simulink model "sampleModel365"  (R2021b)
settings: Solver=VariableStepAuto  StartTime=0.0  StopTime=10.0  RelTol=1e-3
undefined symbols (not defined in the file or in its folder): DiscIntNeverNeededParam
libraries: simulink x9, slpidlib x4
settings Model: Creator=user  LastModifiedBy=user

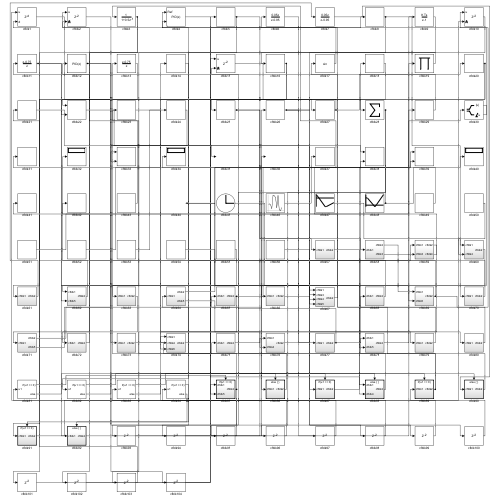
[thumbnail: Simulink's stored preview of the top-level diagram]
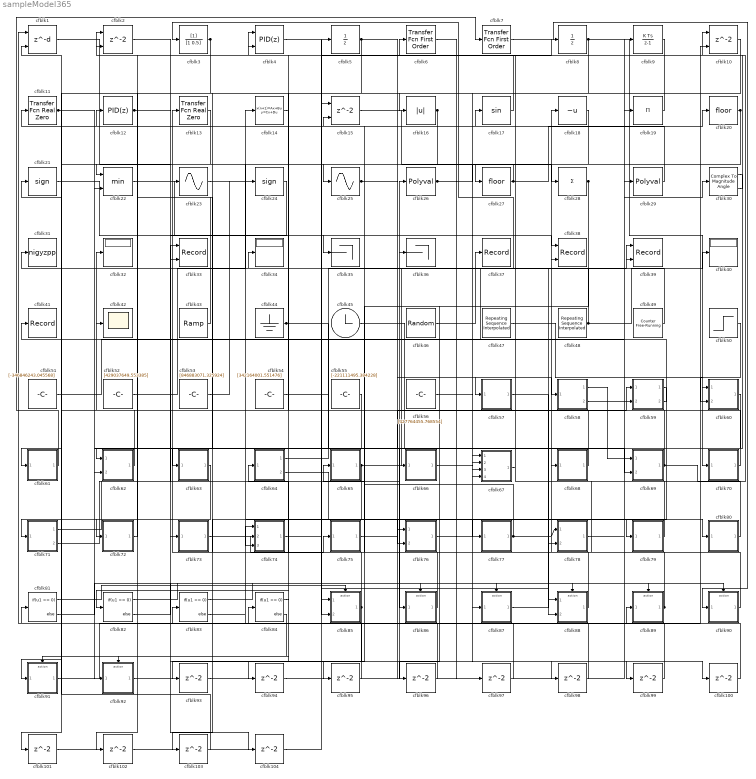
== system sampleModel365 ==
  cfblk1 : Delay  DelayLengthSource=Input port  SampleTime=1
      settings: InputPortMap=u0,p1
  cfblk10 : Delay  ShowEnablePort=on  SampleTime=1
      settings: InputPortMap=u0,e6
  cfblk{93..104} (12 alike) : Delay  SampleTime=1
  cfblk11 : simulink/Discrete/Transfer Fcn Real Zero  ZeroZ=0.75  ICPrevInput=0.0  DoSatur=off
      settings: SourceProductBaseCode=SL
  cfblk12 : slpidlib/PID Controller  Controller=PID  Form=Parallel  TimeDomain=Discrete-time  UseExternalTs=off  SampleTime=1  IntegratorMethod=Forward Euler  FilterMethod=Forward Euler  ControllerParametersSource=internal  P=1  I=1  D=0  UseFilter=on  N=100  TunerSelectOption=Transfer Function Based (PID Tuner App)  InitialConditionSource=internal  InitialConditionForIntegrator=0  InitialConditionForFilter=0  DifferentiatorICPrevScaledInput=0  ExternalReset=none  TrackingMode=off  Kt=1  LimitOutput=off  SatLimitsSource=internal  UpperSaturationLimit=inf  LowerSaturationLimit=-inf  LinearizeAsGain=off  AntiWindupMode=none  Kb=1  POutMin=[]  POutMax=[]  IOutMin=[]  IOutMax=[]  DOutMin=[]  DOutMax=[]  NOutMin=[]  NOutMax=[]  SumOutMin=[]  SumOutMax=[]  SaturationOutMin=[]  SaturationOutMax=[]  PParamMin=[]  PParamMax=[]  IParamMin=[]  IParamMax=[]  DParamMin=[]  DParamMax=[]  NParamMin=[]  NParamMax=[]  KbParamMin=[]  KbParamMax=[]  KtParamMin=[]  KtParamMax=[]  KbOutMin=[]  KbOutMax=[]  KtOutMin=[]  KtOutMax=[]  IntegratorOutMin=[]  IntegratorOutMax=[]  FilterOutMin=[]  FilterOutMax=[]  SumI1OutMin=[]  SumI1OutMax=[]  SumI2OutMin=[]  SumI2OutMax=[]  SumI3OutMin=[]  SumI3OutMax=[]  SumI4OutMin=[]  SumI4OutMax=[]  SumDOutMin=[]  SumDOutMax=[]  DifferentiatorOutMin=[]  DifferentiatorOutMax=[]  FilterDiffOutCoefMin=[]  FilterDiffOutCoefMax=[]  ReciprocalOutMin=[]  ReciprocalOutMax=[]  SumDenOutMin=[]  SumDenOutMax=[]  SumNumOutMin=[]  SumNumOutMax=[]  DivideOutMin=[]  DivideOutMax=[]  UdiffTsProdOutMin=[]  UdiffTsProdOutMax=[]  NTsProdOutMin=[]  NTsProdOutMax=[]  UintegralTsProdOutMin=[]  UintegralTsProdOutMax=[]  UngainTsProdOutMin=[]  UngainTsProdOutMax=[]  IntegratorContinuousStateAttributes=''  IntegratorStateMustResolveToSignalObject=off  IntegratorRTWStateStorageClass=Auto  FilterContinuousStateAttributes=''  FilterStateMustResolveToSignalObject=off  FilterRTWStateStorageClass=Auto  ParallelPVariant=InternalParameters  IdealPVariant=Disabled  IVariant=InternalParameters  DVariant=InternalParameters  IntegratorVariant=Discrete  SatVariant=Disabled  AWVariant=Passthrough  PCopyVariant=Disabled  TRVariant=Disabled  FdbkBlocksVariant=Forward  IdealPFdbkVariant=Disabled  SatFdbkVariant=Disabled  DerivativeFilterVariant=ForwardEulerFilter  NVariant=InternalParameters  NCopyVariant=Disabled  FilterICVariant=InternalICsFilter  IntegratorICVariant=InternalICs  ExternalResetVariant=Disabled  TRSumVariant=Passthrough  SumFdbkVariant=Disabled  SumVariant=Sum_PID  TsampFilterVariant=InternalTs  TsampNgainVariant=Passthrough  TsampIntegralVariant=Passthrough  ExternalSaturationOutDataTypeStr=Inherit: Same as second input
  cfblk13 : simulink/Discrete/Transfer Fcn Real Zero  ZeroZ=0.75  ICPrevInput=0.0  DoSatur=off
      settings: SourceProductBaseCode=SL
  cfblk14 : DiscreteStateSpace
  cfblk15 : Delay  ShowEnablePort=on  SampleTime=1
      settings: InputPortMap=u0,e6
  cfblk16 : Abs
  cfblk17 : Trigonometry
  cfblk18 : UnaryMinus
  cfblk19 : Product  Inputs=*
  cfblk2 : Delay  ShowEnablePort=on  SampleTime=1
      settings: InputPortMap=u0,e6
  cfblk20 : Rounding
  cfblk21 : Signum
  cfblk22 : MinMax  Inputs=2
  cfblk23 : Sin  TimeSource=Use external signal  SampleTime=0
  cfblk24 : Signum
  cfblk25 : Sin  TimeSource=Use external signal  SampleTime=0
  cfblk26 : Polyval  Coefs=[ +2.081618890e-019, -1.441693666e-014, +4.719686976e-010, -8.536869453e-006, +1.621573104e-001, -8.087801117e+001 ]
  cfblk27 : Rounding
  cfblk28 : Sum  Inputs=+
  cfblk29 : Polyval  Coefs=[ +2.081618890e-019, -1.441693666e-014, +4.719686976e-010, -8.536869453e-006, +1.621573104e-001, -8.087801117e+001 ]
  cfblk3 : DiscreteFilter  SampleTime=1
  cfblk30 : ComplexToMagnitudeAngle
  cfblk31 : ToWorkspace  VariableName=nigyzpp  SaveFormat=Timeseries  SampleTime=-1
  cfblk32 : Display
  cfblk33 : Record  FileSettingsInternal="{\"entries\":[{\"content\":{\"excelSettings\":{\"content\":{},\"type\":\"Streamout.ExcelSettings\"}},\"type\":\"Streamout.FileSettingStorage\",\"uuid\":\"567b8140-eb5c-4048-b530-8f92b88b9877\"}],\"packageUris\":[\"http://schema.mathworks.com/mf0/streamout_blocks/R2020a\"],\"version\":\"1.0\"}"  Layout=[1 1]  SignalsInternal="{\"entries\":[{\"content\":{\"signals\":[{\"content\":{\"blockPath\":[\"sampleModel365/cfblk33\"],\"channel\":[],\"dimensions\":[1],\"domain\":\"sampleModel365/cfblk33\",\"lineColor\":\"#a2142f\",\"plots\":[1],\"port\":1,\"sid\":[\"\"],\"signalID\":15095,\"signalName\":\"cfblk71:1\"},\"type\":\"RecordBlkView.Signal\",\"uuid\":\"13d7f1e2-b6fb-48eb-b80d-9a015310c975\"},{\"content\":{\"blockPath\":[\"sampleModel365/cfblk33\"],\"channel\":[],\"dimensions\":[1],\"domain\":\"sampleModel365/cfblk33\",\"lineColor\":\"#139fff\",\"plots\":[1],\"port\":2,\"sid\":[\"\"],\"signalID\":15099,\"signalName\":\"cfblk24\"},\"type\":\"RecordBlkView.Signal\",\"uuid\":\"a06a9fc9-9345-432e-829d-64d9e5ba65b8\"}]},\"type\":\"RecordBlkView.InputSignals\",\"uuid\":\"33d499b8-4f10-4db5-961c-bad95c7f5677\"}],\"packageUris\":[\"http://schema.mathworks.com/mf0/streamout_blocks/R2020a\"],\"version\":\"1.0\"}"  VisualizationBindings="{\"xyplotplugin\":{\"info\":[{\"series\":[{\"bindingParametersList\":[{\"parameter\":\"X-Axis\",\"signalID\":15095,\"signalName\":\"cfblk71:1\"},{\"parameter\":\"Y-Axis\",\"signalID\":15099,\"signalName\":\"cfblk24\"}],\"seriesID\":36555}],\"subplotID\":1}]}}"  CompatibilityTag=XY
  cfblk34 : Display
  cfblk35 : Terminator
  cfblk36 : Terminator
  cfblk37 : Record  FileSettingsInternal="{\"entries\":[{\"content\":{\"excelSettings\":{\"content\":{},\"type\":\"Streamout.ExcelSettings\"}},\"type\":\"Streamout.FileSettingStorage\",\"uuid\":\"649bd7b5-baee-4403-bfdf-0451a9d50882\"}],\"packageUris\":[\"http://schema.mathworks.com/mf0/streamout_blocks/R2020a\"],\"version\":\"1.0\"}"  SignalsInternal="{\"entries\":[{\"content\":{\"signals\":[{\"content\":{\"blockPath\":[\"sampleModel365/cfblk37\"],\"channel\":[],\"dimensions\":[1],\"domain\":\"sampleModel365/cfblk37\",\"lineColor\":\"#22b573\",\"plots\":[1],\"port\":1,\"sid\":[\"\"],\"signalID\":15119,\"signalName\":\"cfblk46\"},\"type\":\"RecordBlkView.Signal\",\"uuid\":\"1a7fcce6-5cc4-4007-aa49-3d2bea6aa8b4\"}]},\"type\":\"RecordBlkView.InputSignals\",\"uuid\":\"0982ba8e-6094-4d7a-b36e-3969a046187e\"}],\"packageUris\":[\"http://schema.mathworks.com/mf0/streamout_blocks/R2020a\"],\"version\":\"1.0\"}"  VisualizationBindings="{\"sparklinesplugin\":{\"info\":[{\"bindingParametersList\":[],\"subplotID\":1}]}}"
  cfblk38 : Record  FileSettingsInternal="{\"entries\":[{\"content\":{\"excelSettings\":{\"content\":{},\"type\":\"Streamout.ExcelSettings\"}},\"type\":\"Streamout.FileSettingStorage\",\"uuid\":\"1ff4d437-0c84-40b7-91d9-f5fc12d76050\"}],\"packageUris\":[\"http://schema.mathworks.com/mf0/streamout_blocks/R2020a\"],\"version\":\"1.0\"}"  Layout=[1 1]  SignalsInternal="{\"entries\":[{\"content\":{\"signals\":[{\"content\":{\"blockPath\":[\"sampleModel365/cfblk38\"],\"channel\":[],\"dimensions\":[1],\"domain\":\"sampleModel365/cfblk38\",\"lineColor\":\"#a2142f\",\"plots\":[1],\"port\":1,\"sid\":[\"\"],\"signalID\":15103,\"signalName\":\"cfblk22\"},\"type\":\"RecordBlkView.Signal\",\"uuid\":\"a984cc03-4ad2-4885-a72c-2beb6033d68e\"},{\"content\":{\"blockPath\":[\"sampleModel365/cfblk38\"],\"channel\":[],\"dimensions\":[1],\"domain\":\"sampleModel365/cfblk38\",\"lineColor\":\"#139fff\",\"plots\":[1],\"port\":2,\"sid\":[\"\"],\"signalID\":15123,\"signalName\":\"cfblk44\"},\"type\":\"RecordBlkView.Signal\",\"uuid\":\"cf2bfc31-ea28-4664-8696-6d3ddec068b2\"}]},\"type\":\"RecordBlkView.InputSignals\",\"uuid\":\"835b0b7a-af76-47df-882f-258c594722fd\"}],\"packageUris\":[\"http://schema.mathworks.com/mf0/streamout_blocks/R2020a\"],\"version\":\"1.0\"}"  VisualizationBindings="{\"xyplotplugin\":{\"info\":[{\"series\":[{\"bindingParametersList\":[{\"parameter\":\"X-Axis\",\"signalID\":15103,\"signalName\":\"cfblk22\"},{\"parameter\":\"Y-Axis\",\"signalID\":15123,\"signalName\":\"cfblk44\"}],\"seriesID\":61757}],\"subplotID\":1}]}}"  CompatibilityTag=XY
  cfblk39 : Record  FileSettingsInternal="{\"entries\":[{\"content\":{\"excelSettings\":{\"content\":{},\"type\":\"Streamout.ExcelSettings\"}},\"type\":\"Streamout.FileSettingStorage\",\"uuid\":\"35b5ed4a-cb0b-4459-8fb2-d4d30692ccee\"}],\"packageUris\":[\"http://schema.mathworks.com/mf0/streamout_blocks/R2020a\"],\"version\":\"1.0\"}"  Layout=[1 1]  SignalsInternal="{\"entries\":[{\"content\":{\"signals\":[{\"content\":{\"blockPath\":[\"sampleModel365/cfblk39\"],\"channel\":[],\"dimensions\":[1],\"domain\":\"sampleModel365/cfblk39\",\"lineColor\":\"#a2142f\",\"plots\":[1],\"port\":1,\"sid\":[\"\"],\"signalID\":15107,\"signalName\":\"cfblk65\"},\"type\":\"RecordBlkView.Signal\",\"uuid\":\"c0428a1b-d602-48ef-ba58-3bcf674a13e3\"},{\"content\":{\"blockPath\":[\"sampleModel365/cfblk39\"],\"channel\":[],\"dimensions\":[1],\"domain\":\"sampleModel365/cfblk39\",\"lineColor\":\"#139fff\",\"plots\":[1],\"port\":2,\"sid\":[\"\"],\"signalID\":15111,\"signalName\":\"cfblk87\"},\"type\":\"RecordBlkView.Signal\",\"uuid\":\"106950b7-24c9-4dcc-9644-3f44a9cb415d\"}]},\"type\":\"RecordBlkView.InputSignals\",\"uuid\":\"4c517a09-619e-4c48-972b-e804149b64f6\"}],\"packageUris\":[\"http://schema.mathworks.com/mf0/streamout_blocks/R2020a\"],\"version\":\"1.0\"}"  VisualizationBindings="{\"xyplotplugin\":{\"info\":[{\"series\":[{\"bindingParametersList\":[{\"parameter\":\"X-Axis\",\"signalID\":15107,\"signalName\":\"cfblk65\"},{\"parameter\":\"Y-Axis\",\"signalID\":15111,\"signalName\":\"cfblk87\"}],\"seriesID\":63832}],\"subplotID\":1}]}}"  CompatibilityTag=XY
  cfblk4 : slpidlib/PID Controller (2DOF)  Controller=PID  Form=Parallel  TimeDomain=Discrete-time  UseExternalTs=off  SampleTime=1  IntegratorMethod=Forward Euler  FilterMethod=Forward Euler  ControllerParametersSource=internal  P=1  I=1  D=0  UseFilter=on  N=100  b=1  c=1  TunerSelectOption=Transfer Function Based (PID Tuner App)  InitialConditionSource=internal  InitialConditionForIntegrator=0  InitialConditionForFilter=0  DifferentiatorICPrevScaledInput=0  ExternalReset=none  TrackingMode=off  Kt=1  LimitOutput=off  SatLimitsSource=internal  UpperSaturationLimit=inf  LowerSaturationLimit=-inf  LinearizeAsGain=off  AntiWindupMode=none  Kb=1  POutMin=[]  POutMax=[]  IOutMin=[]  IOutMax=[]  DOutMin=[]  DOutMax=[]  NOutMin=[]  NOutMax=[]  bOutMin=[]  bOutMax=[]  cOutMin=[]  cOutMax=[]  SumOutMin=[]  SumOutMax=[]  SaturationOutMin=[]  SaturationOutMax=[]  PParamMin=[]  PParamMax=[]  IParamMin=[]  IParamMax=[]  DParamMin=[]  DParamMax=[]  NParamMin=[]  NParamMax=[]  bParamMin=[]  bParamMax=[]  cParamMin=[]  cParamMax=[]  KbParamMin=[]  KbParamMax=[]  KtParamMin=[]  KtParamMax=[]  KbOutMin=[]  KbOutMax=[]  KtOutMin=[]  KtOutMax=[]  IntegratorOutMin=[]  IntegratorOutMax=[]  FilterOutMin=[]  FilterOutMax=[]  SumI1OutMin=[]  SumI1OutMax=[]  SumI2OutMin=[]  SumI2OutMax=[]  SumI3OutMin=[]  SumI3OutMax=[]  SumI4OutMin=[]  SumI4OutMax=[]  SumDOutMin=[]  SumDOutMax=[]  Sum1OutMin=[]  Sum1OutMax=[]  Sum2OutMin=[]  Sum2OutMax=[]  Sum3OutMin=[]  Sum3OutMax=[]  DifferentiatorOutMin=[]  DifferentiatorOutMax=[]  FilterDiffOutCoefMin=[]  FilterDiffOutCoefMax=[]  ReciprocalOutMin=[]  ReciprocalOutMax=[]  SumDenOutMin=[]  SumDenOutMax=[]  SumNumOutMin=[]  SumNumOutMax=[]  DivideOutMin=[]  DivideOutMax=[]  UdiffTsProdOutMin=[]  UdiffTsProdOutMax=[]  NTsProdOutMin=[]  NTsProdOutMax=[]  UintegralTsProdOutMin=[]  UintegralTsProdOutMax=[]  UngainTsProdOutMin=[]  UngainTsProdOutMax=[]  IntegratorContinuousStateAttributes=''  IntegratorStateMustResolveToSignalObject=off  IntegratorRTWStateStorageClass=Auto  FilterContinuousStateAttributes=''  FilterStateMustResolveToSignalObject=off  FilterRTWStateStorageClass=Auto  ParallelPVariant=InternalParameters  IdealPVariant=Disabled  IVariant=InternalParameters  DVariant=InternalParameters  bVariant=InternalParameters  cVariant=InternalParameters  IntegratorVariant=Discrete  SatVariant=Disabled  AWVariant=Passthrough  PCopyVariant=Disabled  TRVariant=Disabled  FdbkBlocksVariant=Forward  IdealPFdbkVariant=Disabled  SatFdbkVariant=Disabled  DerivativeFilterVariant=ForwardEulerFilter  NVariant=InternalParameters  NCopyVariant=Disabled  FilterICVariant=InternalICsFilter  IntegratorICVariant=InternalICs  ExternalResetVariant=Disabled  TRSumVariant=Passthrough  SumFdbkVariant=Disabled  SumVariant=Sum_PID  TsampFilterVariant=InternalTs  TsampNgainVariant=Passthrough  TsampIntegralVariant=Passthrough  ExternalSaturationOutDataTypeStr=Inherit: Same as second input
      settings: SourceProductBaseCode=SL
  cfblk40 : Display
  cfblk41 : Record  FileSettingsInternal="{\"entries\":[{\"content\":{\"excelSettings\":{\"content\":{},\"type\":\"Streamout.ExcelSettings\"}},\"type\":\"Streamout.FileSettingStorage\",\"uuid\":\"5481fc23-8463-4565-9524-5e1ed1cb160f\"}],\"packageUris\":[\"http://schema.mathworks.com/mf0/streamout_blocks/R2020a\"],\"version\":\"1.0\"}"  SignalsInternal="{\"entries\":[{\"content\":{\"signals\":[{\"content\":{\"blockPath\":[\"sampleModel365/cfblk41\"],\"channel\":[],\"dimensions\":[1],\"domain\":\"sampleModel365/cfblk41\",\"lineColor\":\"#fe330a\",\"plots\":[1],\"port\":1,\"sid\":[\"\"],\"signalID\":15115,\"signalName\":\"cfblk59:2\"},\"type\":\"RecordBlkView.Signal\",\"uuid\":\"222ed1ed-24d6-4460-972e-87adfa1e83d3\"}]},\"type\":\"RecordBlkView.InputSignals\",\"uuid\":\"1feaa0a2-3980-4dbe-9ab3-42cb594308e1\"}],\"packageUris\":[\"http://schema.mathworks.com/mf0/streamout_blocks/R2020a\"],\"version\":\"1.0\"}"  VisualizationBindings="{\"sparklinesplugin\":{\"info\":[{\"bindingParametersList\":[],\"subplotID\":1}]}}"
  cfblk42 : Scope
  cfblk43 : simulink/Sources/Ramp  slope=[2383.054350]  start=[44.880096]  InitialOutput=[485045.496723]
  cfblk44 : Ground
  cfblk45 : Clock
  cfblk46 : RandomNumber  Mean=[75307.969094]  Variance=[43913.906071]  Seed=[27084174.000000]  SampleTime=0.1
  cfblk47 : simulink/Sources/Repeating Sequence Interpolated  OutValues=[324115040.329646, 113958309.694816, -785240119.694534, -752060174.629684, -422976193.941777]  TimeValues=[0 0.1 0.5 0.6 1].'  LookUpMeth=Use Input Nearest  tsamp=0.01  OutMin=[]  OutMax=[]  OutDataTypeStr=double  OutputDataTypeScalingMode=double  OutDataType=fixdt(0,8)  OutScaling=2^-10
  cfblk48 : simulink/Sources/Repeating Sequence Interpolated  OutValues=[666690424.086203, 616793045.343907, -127611017.511921, 16668326.026093, 946909106.545576]  TimeValues=[0 0.1 0.5 0.6 1].'  LookUpMeth=Use Input Below  tsamp=0.01  OutMin=[]  OutMax=[]  OutDataTypeStr=double  OutputDataTypeScalingMode=double  OutDataType=fixdt(0,8)  OutScaling=2^-10
  cfblk49 : simulink/Sources/Counter Free-Running  NumBits=[29.000000]  tsamp=-1
  cfblk5 : UnitDelay  HasFrameUpgradeWarning=on
  cfblk50 : Step  Time=[41.000000]  Before=[181754476.570915]  After=[944807555.087493]  SampleTime=0
  cfblk51 : Constant  Value=[-346846243.045568]  SampleTime=1
  cfblk52 : Constant  Value=[429037649.553385]  SampleTime=1
  cfblk53 : Constant  Value=[846883071.325924]  SampleTime=1
  cfblk54 : Constant  Value=[342164001.551476]  SampleTime=1
  cfblk55 : Constant  Value=[-221111495.384228]  SampleTime=1
  cfblk56 : Constant  Value=[427764455.768554]  SampleTime=1
  cfblk57 : Subsystem
  cfblk58 : Subsystem
  cfblk59 : Subsystem
  cfblk6 : simulink/Discrete/Transfer Fcn First Order  PoleZ=0.95  ICPrevOutput=0.0  DoSatur=off
  cfblk60 : Subsystem
  cfblk61 : Subsystem
  cfblk62 : Subsystem
  cfblk63 : Subsystem
  cfblk64 : Subsystem
  cfblk65 : Subsystem
  cfblk66 : Subsystem
  cfblk67 : Subsystem
  cfblk68 : Subsystem
  cfblk69 : Subsystem
  cfblk7 : simulink/Discrete/Transfer Fcn First Order  PoleZ=0.95  ICPrevOutput=0.0  DoSatur=off
  cfblk70 : Subsystem
  cfblk71 : Subsystem
  cfblk72 : Subsystem
  cfblk73 : Subsystem
  cfblk74 : Subsystem
  cfblk75 : Subsystem
  cfblk76 : Subsystem
  cfblk77 : Subsystem
  cfblk78 : Subsystem
  cfblk79 : Subsystem
  cfblk8 : UnitDelay  HasFrameUpgradeWarning=on
  cfblk80 : Subsystem
  cfblk{81..84} (4 alike) : If  IfExpression=u1 >= 0  SampleTime=1
  cfblk85 : Subsystem  TreatAsAtomicUnit=on
  cfblk86 : Subsystem  TreatAsAtomicUnit=on
  cfblk87 : Subsystem  TreatAsAtomicUnit=on
  cfblk88 : Subsystem  TreatAsAtomicUnit=on
  cfblk89 : Subsystem  TreatAsAtomicUnit=on
  cfblk9 : DiscreteIntegrator  ICPrevOutput=DiscIntNeverNeededParam  ICPrevScaledInput=DiscIntNeverNeededParam
  cfblk90 : Subsystem  TreatAsAtomicUnit=on
  cfblk91 : Subsystem  TreatAsAtomicUnit=on
  cfblk92 : Subsystem  TreatAsAtomicUnit=on
  wires:
  cfblk89/1(cfblk2) -> cfblk18/1, cfblk68/1(cfblk1)
  cfblk14/1 -> cfblk82/1
  cfblk6/1 -> cfblk77/1(cfblk1)
  cfblk46/1 -> cfblk37/1
  cfblk47/1 -> cfblk70/1(cfblk1)
  cfblk92/1(cfblk2) -> cfblk26/1
  cfblk53/1 -> cfblk24/1
  cfblk67/1(cfblk2) -> cfblk3/1
  cfblk85/1(cfblk2) -> cfblk13/1, cfblk103/1
  cfblk3/1 -> cfblk22/1, cfblk72/1(cfblk1)
  cfblk25/1 -> cfblk58/1(cfblk1), cfblk67/4(cfblk5)
  cfblk5/1 -> cfblk63/1(cfblk1), cfblk57/1(cfblk1)
  cfblk1/1 -> cfblk73/1(cfblk1)
  cfblk58/1(cfblk2) -> cfblk69/1(cfblk1)
  cfblk30/1 -> cfblk62/1(cfblk1)
  cfblk54/1 -> cfblk69/2(cfblk5)
  cfblk60/1(cfblk2) -> cfblk86/1(cfblk1)
  cfblk15/1 -> cfblk27/1
  cfblk55/1 -> cfblk62/2(cfblk5)
  cfblk48/1 -> cfblk34/1, cfblk40/1
  cfblk71/1(cfblk2) -> cfblk33/1
  cfblk71/2(cfblk5) -> cfblk36/1
  cfblk69/1(cfblk2) -> cfblk10/1, cfblk12/1
  cfblk70/1(cfblk2) -> cfblk32/1
  cfblk65/1(cfblk2) -> cfblk39/1, cfblk93/1
  cfblk57/1(cfblk2) -> cfblk88/1(cfblk1)
  cfblk87/1(cfblk2) -> cfblk39/2
  cfblk29/1 -> cfblk17/1
  cfblk23/1 -> cfblk76/2(cfblk4)
  cfblk19/1 -> cfblk16/1
  cfblk49/1 -> cfblk31/1
  cfblk26/1 -> cfblk28/1, cfblk97/1, cfblk98/1
  cfblk21/1 -> cfblk67/1(cfblk1)
  cfblk56/1 -> cfblk87/1(cfblk1)
  cfblk7/1 -> cfblk90/1(cfblk1)
  cfblk18/1 -> cfblk22/2
  cfblk27/1 -> cfblk20/1, cfblk25/1
  cfblk22/1 -> cfblk38/1
  cfblk17/1 -> cfblk6/1
  cfblk4/1 -> cfblk88/2(cfblk4)
  cfblk30/2 -> cfblk4/1
  cfblk91/1(cfblk2) -> cfblk10/2
  cfblk28/1 -> cfblk95/1, cfblk96/1
  cfblk68/1(cfblk2) -> cfblk4/2
  cfblk8/1 -> cfblk60/1(cfblk1), cfblk61/1(cfblk1)
  cfblk44/1 -> cfblk38/2, cfblk67/3(cfblk4)
  cfblk76/1(cfblk2) -> cfblk80/1(cfblk1)
  cfblk62/1(cfblk2) -> cfblk21/1
  cfblk73/1(cfblk2) -> cfblk75/1(cfblk1)
  cfblk75/1(cfblk2) -> cfblk59/1(cfblk1)
  cfblk78/1(cfblk2) -> cfblk9/1
  cfblk43/1 -> cfblk2/1
  cfblk79/1(cfblk2) -> cfblk11/1
  cfblk88/1(cfblk2) -> cfblk64/1(cfblk1)
  cfblk74/1(cfblk2) -> cfblk8/1
  cfblk61/1(cfblk2) -> cfblk7/1
  cfblk90/1(cfblk2) -> cfblk23/1
  cfblk12/1 -> cfblk35/1, cfblk104/1
  cfblk77/1(cfblk2) -> cfblk78/1(cfblk1), cfblk15/2
  cfblk80/1(cfblk2) -> cfblk2/2
  cfblk45/1 -> cfblk78/2(cfblk5)
  cfblk9/1 -> cfblk67/2(cfblk3)
  cfblk16/1 -> cfblk91/1(cfblk1), cfblk71/1(cfblk1)
  cfblk51/1 -> cfblk29/1
  cfblk52/1 -> cfblk14/1
  cfblk64/1(cfblk2) -> cfblk19/1
  cfblk20/1 -> cfblk85/2(cfblk5), cfblk74/3(cfblk5)
  cfblk58/2(cfblk3) -> cfblk30/1
  cfblk59/1(cfblk2) -> cfblk74/2(cfblk4)
  cfblk24/1 -> cfblk33/2
  cfblk59/2(cfblk4) -> cfblk41/1
  cfblk50/1 -> cfblk60/2(cfblk4)
  cfblk86/1(cfblk2) -> cfblk65/1(cfblk1)
  cfblk11/1 -> cfblk92/1(cfblk1), cfblk66/1(cfblk1)
  cfblk72/1(cfblk2) -> cfblk42/1
  cfblk64/2(cfblk5) -> cfblk79/1(cfblk1)
  cfblk81/1 -> cfblk85/Action
  cfblk81/2 -> cfblk86/Action
  cfblk82/1 -> cfblk87/Action
  cfblk82/2 -> cfblk88/Action
  cfblk83/1 -> cfblk89/Action
  cfblk83/2 -> cfblk90/Action
  cfblk84/1 -> cfblk91/Action
  cfblk84/2 -> cfblk92/Action
  cfblk93/1 -> cfblk59/2(cfblk3)
  cfblk10/1 -> cfblk94/1
  cfblk94/1 -> cfblk76/1(cfblk1)
  cfblk95/1 -> cfblk74/1(cfblk1)
  cfblk96/1 -> cfblk1/1
  cfblk97/1 -> cfblk1/2
  cfblk98/1 -> cfblk84/1
  cfblk66/1(cfblk2) -> cfblk99/1
  cfblk99/1 -> cfblk89/1(cfblk1)
  cfblk2/1 -> cfblk100/1
  cfblk100/1 -> cfblk83/1
  cfblk63/1(cfblk2) -> cfblk101/1
  cfblk101/1 -> cfblk5/1
  cfblk13/1 -> cfblk102/1
  cfblk102/1 -> cfblk85/1(cfblk1)
  cfblk103/1 -> cfblk81/1
  cfblk104/1 -> cfblk15/1

== system sampleModel365/cfblk57 ==
  cfblk1 : Inport
  cfblk3 : DiscreteTransferFcn  SampleTime=1
  cfblk2 : Outport
  wires:
  cfblk1/1 -> cfblk3/1
  cfblk3/1 -> cfblk2/1

== system sampleModel365/cfblk58 ==
  cfblk1 : Inport
  cfblk2 : Outport
  cfblk3 : Outport  Port=2
  wires:
  cfblk1/1 -> cfblk3/1, cfblk2/1

== system sampleModel365/cfblk59 ==
  cfblk1 : Inport
  cfblk3 : Inport  Port=2
  cfblk2 : Outport
  cfblk4 : Outport  Port=2
  wires:
  cfblk3/1 -> cfblk2/1
  cfblk1/1 -> cfblk4/1

== system sampleModel365/cfblk60 ==
  cfblk1 : Inport
  cfblk4 : Inport  Port=2
  cfblk3 : Bias  Bias=[-14351574.629896]
  cfblk2 : Outport
  wires:
  cfblk1/1 -> cfblk3/1
  cfblk3/1 -> cfblk2/1

== system sampleModel365/cfblk61 ==
  cfblk1 : Inport
  cfblk3 : MinMax  Inputs=2
  cfblk2 : Outport
  wires:
  cfblk3/1 -> cfblk2/1
  cfblk1/1 -> cfblk3/1, cfblk3/2

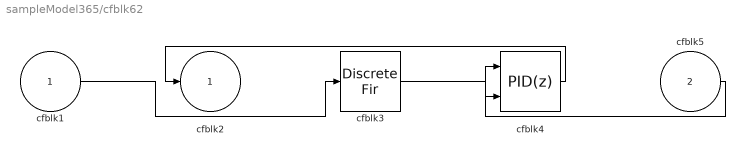
== system sampleModel365/cfblk62 ==
  cfblk1 : Inport
  cfblk5 : Inport  Port=2
  cfblk3 : DiscreteFir  SampleTime=1
  cfblk4 : slpidlib/PID Controller (2DOF)  Controller=PID  Form=Parallel  TimeDomain=Discrete-time  UseExternalTs=off  SampleTime=1  IntegratorMethod=Forward Euler  FilterMethod=Forward Euler  ControllerParametersSource=internal  P=1  I=1  D=0  UseFilter=on  N=100  b=1  c=1  TunerSelectOption=Transfer Function Based (PID Tuner App)  InitialConditionSource=internal  InitialConditionForIntegrator=0  InitialConditionForFilter=0  DifferentiatorICPrevScaledInput=0  ExternalReset=none  TrackingMode=off  Kt=1  LimitOutput=off  SatLimitsSource=internal  UpperSaturationLimit=inf  LowerSaturationLimit=-inf  LinearizeAsGain=off  AntiWindupMode=none  Kb=1  POutMin=[]  POutMax=[]  IOutMin=[]  IOutMax=[]  DOutMin=[]  DOutMax=[]  NOutMin=[]  NOutMax=[]  bOutMin=[]  bOutMax=[]  cOutMin=[]  cOutMax=[]  SumOutMin=[]  SumOutMax=[]  SaturationOutMin=[]  SaturationOutMax=[]  PParamMin=[]  PParamMax=[]  IParamMin=[]  IParamMax=[]  DParamMin=[]  DParamMax=[]  NParamMin=[]  NParamMax=[]  bParamMin=[]  bParamMax=[]  cParamMin=[]  cParamMax=[]  KbParamMin=[]  KbParamMax=[]  KtParamMin=[]  KtParamMax=[]  KbOutMin=[]  KbOutMax=[]  KtOutMin=[]  KtOutMax=[]  IntegratorOutMin=[]  IntegratorOutMax=[]  FilterOutMin=[]  FilterOutMax=[]  SumI1OutMin=[]  SumI1OutMax=[]  SumI2OutMin=[]  SumI2OutMax=[]  SumI3OutMin=[]  SumI3OutMax=[]  SumI4OutMin=[]  SumI4OutMax=[]  SumDOutMin=[]  SumDOutMax=[]  Sum1OutMin=[]  Sum1OutMax=[]  Sum2OutMin=[]  Sum2OutMax=[]  Sum3OutMin=[]  Sum3OutMax=[]  DifferentiatorOutMin=[]  DifferentiatorOutMax=[]  FilterDiffOutCoefMin=[]  FilterDiffOutCoefMax=[]  ReciprocalOutMin=[]  ReciprocalOutMax=[]  SumDenOutMin=[]  SumDenOutMax=[]  SumNumOutMin=[]  SumNumOutMax=[]  DivideOutMin=[]  DivideOutMax=[]  UdiffTsProdOutMin=[]  UdiffTsProdOutMax=[]  NTsProdOutMin=[]  NTsProdOutMax=[]  UintegralTsProdOutMin=[]  UintegralTsProdOutMax=[]  UngainTsProdOutMin=[]  UngainTsProdOutMax=[]  IntegratorContinuousStateAttributes=''  IntegratorStateMustResolveToSignalObject=off  IntegratorRTWStateStorageClass=Auto  FilterContinuousStateAttributes=''  FilterStateMustResolveToSignalObject=off  FilterRTWStateStorageClass=Auto  ParallelPVariant=InternalParameters  IdealPVariant=Disabled  IVariant=InternalParameters  DVariant=InternalParameters  bVariant=InternalParameters  cVariant=InternalParameters  IntegratorVariant=Discrete  SatVariant=Disabled  AWVariant=Passthrough  PCopyVariant=Disabled  TRVariant=Disabled  FdbkBlocksVariant=Forward  IdealPFdbkVariant=Disabled  SatFdbkVariant=Disabled  DerivativeFilterVariant=ForwardEulerFilter  NVariant=InternalParameters  NCopyVariant=Disabled  FilterICVariant=InternalICsFilter  IntegratorICVariant=InternalICs  ExternalResetVariant=Disabled  TRSumVariant=Passthrough  SumFdbkVariant=Disabled  SumVariant=Sum_PID  TsampFilterVariant=InternalTs  TsampNgainVariant=Passthrough  TsampIntegralVariant=Passthrough  ExternalSaturationOutDataTypeStr=Inherit: Same as second input
      settings: SourceProductBaseCode=SL
  cfblk2 : Outport
  wires:
  cfblk4/1 -> cfblk2/1
  cfblk1/1 -> cfblk3/1
  cfblk5/1 -> cfblk4/1
  cfblk3/1 -> cfblk4/2

== system sampleModel365/cfblk63 ==
  cfblk1 : Inport
  cfblk3 : DiscreteZeroPole  Poles=[0 0.5]  Gain=1
  cfblk2 : Outport
  wires:
  cfblk3/1 -> cfblk2/1
  cfblk1/1 -> cfblk3/1

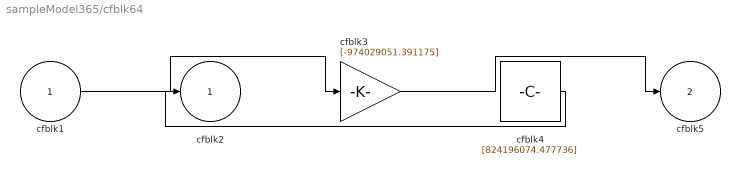
== system sampleModel365/cfblk64 ==
  cfblk1 : Inport
  cfblk3 : Gain  Gain=[-974029051.391175]
  cfblk4 : Constant  Value=[824196074.477736]  SampleTime=1
  cfblk2 : Outport
  cfblk5 : Outport  Port=2
  wires:
  cfblk1/1 -> cfblk3/1
  cfblk3/1 -> cfblk5/1
  cfblk4/1 -> cfblk2/1

== system sampleModel365/cfblk65 ==
  cfblk1 : Inport
  cfblk3 : DiscreteFilter  SampleTime=1
  cfblk4 : Sum  Inputs=+-
  cfblk2 : Outport
  wires:
  cfblk1/1 -> cfblk3/1, cfblk4/2
  cfblk3/1 -> cfblk4/1
  cfblk4/1 -> cfblk2/1

== system sampleModel365/cfblk66 ==
  cfblk1 : Inport
  cfblk3 : Sin  TimeSource=Use external signal  SampleTime=0
  cfblk2 : Outport
  wires:
  cfblk1/1 -> cfblk3/1
  cfblk3/1 -> cfblk2/1

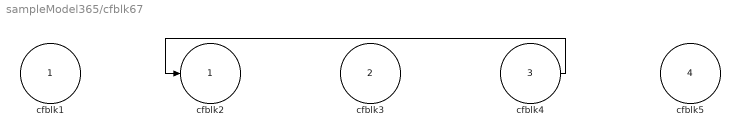
== system sampleModel365/cfblk67 ==
  cfblk1 : Inport
  cfblk3 : Inport  Port=2
  cfblk4 : Inport  Port=3
  cfblk5 : Inport  Port=4
  cfblk2 : Outport
  wires:
  cfblk4/1 -> cfblk2/1

== system sampleModel365/cfblk68 ==
  cfblk1 : Inport
  cfblk3 : slpidlib/PID Controller (2DOF)  Controller=PID  Form=Parallel  TimeDomain=Discrete-time  UseExternalTs=off  SampleTime=1  IntegratorMethod=Forward Euler  FilterMethod=Forward Euler  ControllerParametersSource=internal  P=1  I=1  D=0  UseFilter=on  N=100  b=1  c=1  TunerSelectOption=Transfer Function Based (PID Tuner App)  InitialConditionSource=internal  InitialConditionForIntegrator=0  InitialConditionForFilter=0  DifferentiatorICPrevScaledInput=0  ExternalReset=none  TrackingMode=off  Kt=1  LimitOutput=off  SatLimitsSource=internal  UpperSaturationLimit=inf  LowerSaturationLimit=-inf  LinearizeAsGain=off  AntiWindupMode=none  Kb=1  POutMin=[]  POutMax=[]  IOutMin=[]  IOutMax=[]  DOutMin=[]  DOutMax=[]  NOutMin=[]  NOutMax=[]  bOutMin=[]  bOutMax=[]  cOutMin=[]  cOutMax=[]  SumOutMin=[]  SumOutMax=[]  SaturationOutMin=[]  SaturationOutMax=[]  PParamMin=[]  PParamMax=[]  IParamMin=[]  IParamMax=[]  DParamMin=[]  DParamMax=[]  NParamMin=[]  NParamMax=[]  bParamMin=[]  bParamMax=[]  cParamMin=[]  cParamMax=[]  KbParamMin=[]  KbParamMax=[]  KtParamMin=[]  KtParamMax=[]  KbOutMin=[]  KbOutMax=[]  KtOutMin=[]  KtOutMax=[]  IntegratorOutMin=[]  IntegratorOutMax=[]  FilterOutMin=[]  FilterOutMax=[]  SumI1OutMin=[]  SumI1OutMax=[]  SumI2OutMin=[]  SumI2OutMax=[]  SumI3OutMin=[]  SumI3OutMax=[]  SumI4OutMin=[]  SumI4OutMax=[]  SumDOutMin=[]  SumDOutMax=[]  Sum1OutMin=[]  Sum1OutMax=[]  Sum2OutMin=[]  Sum2OutMax=[]  Sum3OutMin=[]  Sum3OutMax=[]  DifferentiatorOutMin=[]  DifferentiatorOutMax=[]  FilterDiffOutCoefMin=[]  FilterDiffOutCoefMax=[]  ReciprocalOutMin=[]  ReciprocalOutMax=[]  SumDenOutMin=[]  SumDenOutMax=[]  SumNumOutMin=[]  SumNumOutMax=[]  DivideOutMin=[]  DivideOutMax=[]  UdiffTsProdOutMin=[]  UdiffTsProdOutMax=[]  NTsProdOutMin=[]  NTsProdOutMax=[]  UintegralTsProdOutMin=[]  UintegralTsProdOutMax=[]  UngainTsProdOutMin=[]  UngainTsProdOutMax=[]  IntegratorContinuousStateAttributes=''  IntegratorStateMustResolveToSignalObject=off  IntegratorRTWStateStorageClass=Auto  FilterContinuousStateAttributes=''  FilterStateMustResolveToSignalObject=off  FilterRTWStateStorageClass=Auto  ParallelPVariant=InternalParameters  IdealPVariant=Disabled  IVariant=InternalParameters  DVariant=InternalParameters  bVariant=InternalParameters  cVariant=InternalParameters  IntegratorVariant=Discrete  SatVariant=Disabled  AWVariant=Passthrough  PCopyVariant=Disabled  TRVariant=Disabled  FdbkBlocksVariant=Forward  IdealPFdbkVariant=Disabled  SatFdbkVariant=Disabled  DerivativeFilterVariant=ForwardEulerFilter  NVariant=InternalParameters  NCopyVariant=Disabled  FilterICVariant=InternalICsFilter  IntegratorICVariant=InternalICs  ExternalResetVariant=Disabled  TRSumVariant=Passthrough  SumFdbkVariant=Disabled  SumVariant=Sum_PID  TsampFilterVariant=InternalTs  TsampNgainVariant=Passthrough  TsampIntegralVariant=Passthrough  ExternalSaturationOutDataTypeStr=Inherit: Same as second input
      settings: SourceProductBaseCode=SL
  cfblk4 : Reshape
  cfblk2 : Outport
  wires:
  cfblk4/1 -> cfblk2/1, cfblk3/2
  cfblk1/1 -> cfblk4/1, cfblk3/1

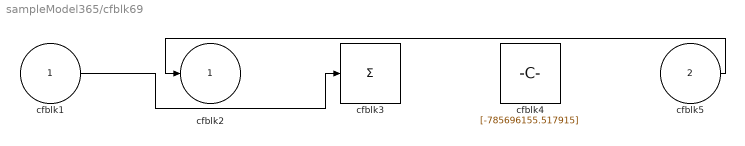
== system sampleModel365/cfblk69 ==
  cfblk1 : Inport
  cfblk5 : Inport  Port=2
  cfblk3 : Sum  Inputs=+
  cfblk4 : Constant  Value=[-785696155.517915]  SampleTime=1
  cfblk2 : Outport
  wires:
  cfblk5/1 -> cfblk2/1
  cfblk1/1 -> cfblk3/1

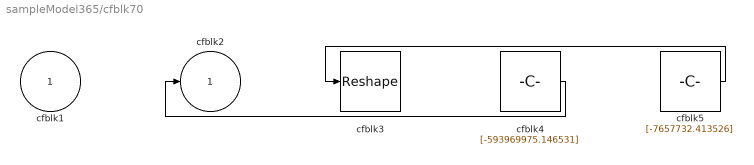
== system sampleModel365/cfblk70 ==
  cfblk1 : Inport
  cfblk3 : Reshape
  cfblk4 : Constant  Value=[-593969975.146531]  SampleTime=1
  cfblk5 : Constant  Value=[-7657732.413526]  SampleTime=1
  cfblk2 : Outport
  wires:
  cfblk5/1 -> cfblk3/1
  cfblk4/1 -> cfblk2/1

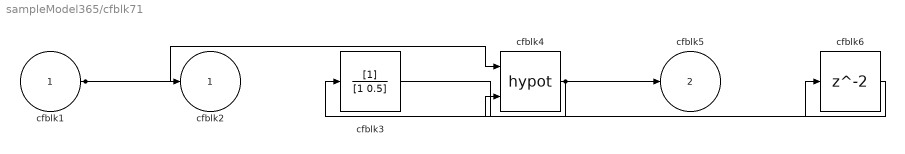
== system sampleModel365/cfblk71 ==
  cfblk1 : Inport
  cfblk3 : DiscreteFilter  SampleTime=1
  cfblk4 : Math  Operator=hypot  SaturateOnIntegerOverflow=on
  cfblk6 : Delay  SampleTime=1
  cfblk2 : Outport
  cfblk5 : Outport  Port=2
  wires:
  cfblk1/1 -> cfblk4/1, cfblk2/1
  cfblk4/1 -> cfblk3/1, cfblk5/1
  cfblk3/1 -> cfblk6/1
  cfblk6/1 -> cfblk4/2

== system sampleModel365/cfblk72 ==
  cfblk1 : Inport
  cfblk3 : Sum  Inputs=|++
  cfblk2 : Outport
  wires:
  cfblk3/1 -> cfblk2/1
  cfblk1/1 -> cfblk3/1, cfblk3/2

== system sampleModel365/cfblk73 ==
  cfblk1 : Inport
  cfblk3 : Constant  Value=[-676484418.441808]  SampleTime=1
  cfblk2 : Outport
  wires:
  cfblk1/1 -> cfblk2/1

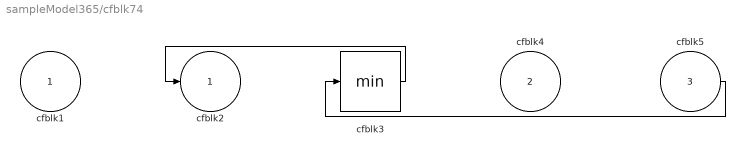
== system sampleModel365/cfblk74 ==
  cfblk1 : Inport
  cfblk4 : Inport  Port=2
  cfblk5 : Inport  Port=3
  cfblk3 : MinMax
  cfblk2 : Outport
  wires:
  cfblk3/1 -> cfblk2/1
  cfblk5/1 -> cfblk3/1

== system sampleModel365/cfblk75 ==
  cfblk1 : Inport
  cfblk3 : DiscreteStateSpace
  cfblk2 : Outport
  wires:
  cfblk1/1 -> cfblk2/1, cfblk3/1

== system sampleModel365/cfblk76 ==
  cfblk1 : Inport
  cfblk4 : Inport  Port=2
  cfblk3 : PermuteDimensions
  cfblk2 : Outport
  wires:
  cfblk4/1 -> cfblk3/1
  cfblk3/1 -> cfblk2/1

== system sampleModel365/cfblk77 ==
  cfblk1 : Inport
  cfblk3 : MinMax  Function=max
  cfblk2 : Outport
  wires:
  cfblk3/1 -> cfblk2/1
  cfblk1/1 -> cfblk3/1

== system sampleModel365/cfblk78 ==
  cfblk1 : Inport
  cfblk5 : Inport  Port=2
  cfblk3 : DiscreteFilter  SampleTime=1
  cfblk4 : UnaryMinus
  cfblk2 : Outport
  wires:
  cfblk1/1 -> cfblk3/1
  cfblk4/1 -> cfblk2/1
  cfblk3/1 -> cfblk4/1

== system sampleModel365/cfblk79 ==
  cfblk1 : Inport
  cfblk3 : Abs
  cfblk4 : Constant  Value=[-342818389.101165]  SampleTime=1
  cfblk2 : Outport
  wires:
  cfblk4/1 -> cfblk3/1
  cfblk1/1 -> cfblk2/1

== system sampleModel365/cfblk80 ==
  cfblk1 : Inport
  cfblk3 : Delay  ShowEnablePort=on  SampleTime=1
      settings: InputPortMap=u0,e6
  cfblk4 : Delay  SampleTime=1
  cfblk5 : Delay  SampleTime=1
  cfblk2 : Outport
  wires:
  cfblk1/1 -> cfblk3/1
  cfblk3/1 -> cfblk4/1
  cfblk4/1 -> cfblk2/1, cfblk5/1
  cfblk5/1 -> cfblk3/2

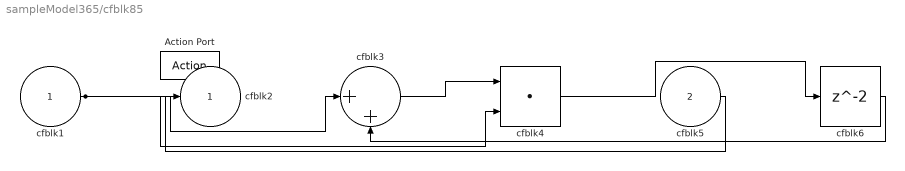
== system sampleModel365/cfblk85 ==
  cfblk1 : Inport
  cfblk5 : Inport  Port=2
  Action Port : ActionPort  ActionPortLabel=if(u1 >= 0)
  cfblk3 : Sum  Inputs=|++
  cfblk4 : DotProduct  InputSameDT=on  OutDataTypeStr=Inherit: Inherit via internal rule
  cfblk6 : Delay
  cfblk2 : Outport
  wires:
  cfblk1/1 -> cfblk3/1, cfblk4/2
  cfblk5/1 -> cfblk2/1
  cfblk3/1 -> cfblk4/1
  cfblk4/1 -> cfblk6/1
  cfblk6/1 -> cfblk3/2

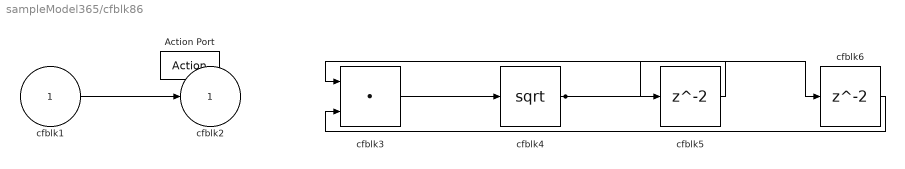
== system sampleModel365/cfblk86 ==
  cfblk1 : Inport
  Action Port : ActionPort  ActionPortLabel=else
  cfblk3 : DotProduct  InputSameDT=on  OutDataTypeStr=Inherit: Inherit via internal rule
  cfblk4 : Sqrt  SaturateOnIntegerOverflow=on
  cfblk5 : Delay
  cfblk6 : Delay
  cfblk2 : Outport
  wires:
  cfblk3/1 -> cfblk4/1
  cfblk1/1 -> cfblk2/1
  cfblk4/1 -> cfblk5/1, cfblk6/1
  cfblk5/1 -> cfblk3/1
  cfblk6/1 -> cfblk3/2

== system sampleModel365/cfblk87 ==
  cfblk1 : Inport
  Action Port : ActionPort  ActionPortLabel=if(u1 >= 0)
  cfblk3 : Sqrt  SaturateOnIntegerOverflow=on
  cfblk2 : Outport
  wires:
  cfblk1/1 -> cfblk2/1, cfblk3/1

== system sampleModel365/cfblk88 ==
  cfblk1 : Inport
  cfblk4 : Inport  Port=2
  Action Port : ActionPort  ActionPortLabel=else
  cfblk3 : Constant  Value=[-230879853.875819]  SampleTime=1
  cfblk2 : Outport
  wires:
  cfblk1/1 -> cfblk2/1

== system sampleModel365/cfblk89 ==
  cfblk1 : Inport
  Action Port : ActionPort  ActionPortLabel=if(u1 >= 0)
  cfblk3 : MinMax  Function=max  Inputs=2
  cfblk2 : Outport
  wires:
  cfblk1/1 -> cfblk3/1, cfblk3/2
  cfblk3/1 -> cfblk2/1

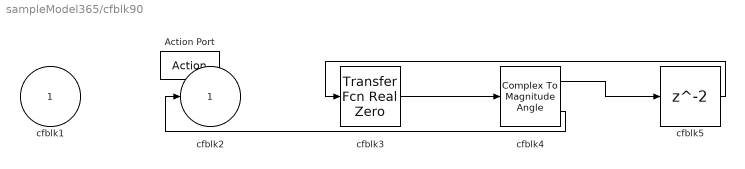
== system sampleModel365/cfblk90 ==
  cfblk1 : Inport
  Action Port : ActionPort  ActionPortLabel=else
  cfblk3 : simulink/Discrete/Transfer Fcn Real Zero  ZeroZ=0.75  ICPrevInput=0.0  DoSatur=off
      settings: SourceProductBaseCode=SL
  cfblk4 : ComplexToMagnitudeAngle
  cfblk5 : Delay
  cfblk2 : Outport
  wires:
  cfblk4/2 -> cfblk2/1
  cfblk3/1 -> cfblk4/1
  cfblk4/1 -> cfblk5/1
  cfblk5/1 -> cfblk3/1

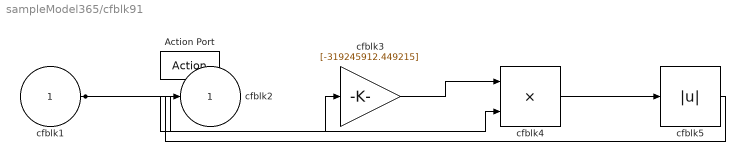
== system sampleModel365/cfblk91 ==
  cfblk1 : Inport
  Action Port : ActionPort  ActionPortLabel=if(u1 >= 0)
  cfblk3 : Gain  Gain=[-319245912.449215]
  cfblk4 : Product  Inputs=**
  cfblk5 : Abs
  cfblk2 : Outport
  wires:
  cfblk3/1 -> cfblk4/1
  cfblk1/1 -> cfblk4/2, cfblk3/1
  cfblk4/1 -> cfblk5/1
  cfblk5/1 -> cfblk2/1

== system sampleModel365/cfblk92 ==
  cfblk1 : Inport
  Action Port : ActionPort  ActionPortLabel=else
  cfblk3 : Sum  Inputs=+
  cfblk2 : Outport
  wires:
  cfblk3/1 -> cfblk2/1
  cfblk1/1 -> cfblk3/1
